simulink model "Timers_Basic"  (R2024a)
settings: Solver=VariableStepAuto  StartTime=0.0  StopTime=10.0  RelTol=1e-3
undefined symbols (not defined in the file or in its folder): DINT, slplc
(part 1 of 2)
settings Model: PacingRate=13  Creator=Jack Vranicar  LastModifiedBy=Jack Vranicar

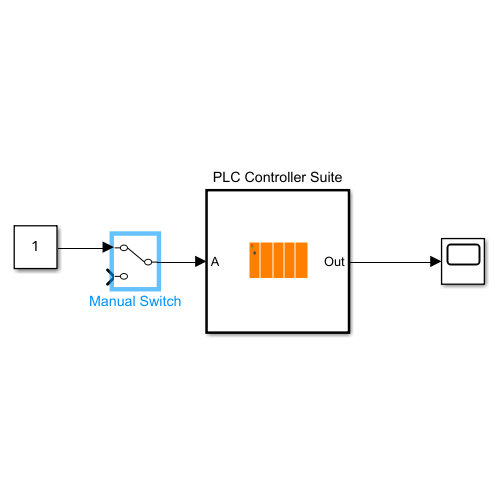
[thumbnail: Simulink's stored preview of the top-level diagram]
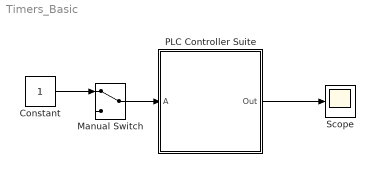
== system Timers_Basic ==
  Constant : Constant  OutDataTypeStr=Inherit: Inherit via back propagation
  Manual Switch : ManualSwitch
  PLC Controller Suite : Subsystem  TreatAsAtomicUnit=on  mask{PLCBlockType=PLCController, PLCPOUType=PLC Controller}
      mask init:
      | slplc.callbacks.initController(gcb);
      settings: OpenFcn=slplc.callbacks.openPOUBlock(gcb);
      mask Help: web([docroot '/plccoder/ref/plccontrollersuite' '.html']);
      mask DialogControl PLCBlockTitle Prompt: PLC Controller Block
  Scope : Scope
  wires:
  Manual Switch/1 -> PLC Controller Suite/1(A)
  Constant/1 -> Manual Switch/1
  PLC Controller Suite/1(Out) -> Scope/1

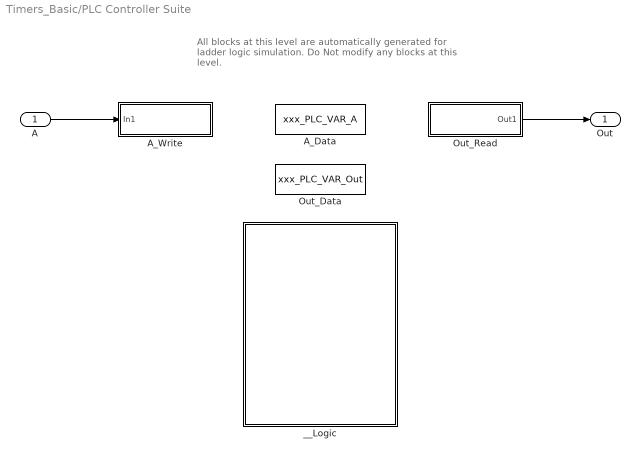
== system Timers_Basic/PLC Controller Suite ==
  note: All blocks at this level are automatically generated for ladder logic simulation.
      | Do Not modify any blocks at this level.
  A : Inport  OutDataTypeStr=boolean
  A_Data : DataStoreMemory  Tag=POUVariable  Priority=10  DataStoreName=xxx_PLC_VAR_A  ShowAdditionalParam=off  OutDataTypeStr=boolean  Dimensions=1
  A_Write : Subsystem  Priority=11  DisableCoverage=on  TreatAsAtomicUnit=on  mask{PLCOperandTag=A, PLCOperandExpression=xxx_PLC_VAR_A, PLCBlockType=VarWrite, PLCPOUType=VarWrite}
      mask prompts: PLCOperandTag "Operand Tag:"
      mask init:
      | slplc.callbacks.initInstruction(gcb);
      mask Help: web([docroot '/plccoder/ref/varwrite' '.html']);
      mask DialogControl PLCBlockTitle Prompt: Variable Write
      mask Display: disp(get_param(gcb, 'PLCOperandTag'));
  Out_Data : DataStoreMemory  Tag=POUVariable  Priority=10  DataStoreName=xxx_PLC_VAR_Out  ShowAdditionalParam=off  OutDataTypeStr=boolean  Dimensions=1
  Out_Read : Subsystem  Priority=13  DisableCoverage=on  TreatAsAtomicUnit=on  mask{PLCOperandTag=Out, PLCOperandExpression=xxx_PLC_VAR_Out, PLCBlockType=VarRead, PLCPOUType=VarRead}
      mask prompts: PLCOperandTag "Operand Tag"
      mask init:
      | block = gcb;
      | maskObj = Simulink.Mask.get(block);
      | maskObj.Display = sprintf('disp(''%s'');', PLCOperandTag);
      | slplc.callbacks.initInstruction(gcb);
      mask Help: web([docroot '/plccoder/ref/varread' '.html']);
      mask DialogControl PLCBlockTitle Prompt: Variable Read
      mask Display: disp('Out');
  __Logic : Subsystem  Priority=12  TreatAsAtomicUnit=on
  Out : Outport
  wires:
  A/1 -> A_Write/1(In1)
  Out_Read/1(Out1) -> Out/1

== system Timers_Basic/PLC Controller Suite/A_Write ==
  In1 : Inport
  __CoreVarWrite : Subsystem  Tag=CoreVarWriteBlock  DisableCoverage=on  TreatAsAtomicUnit=on  mask{PLCBlockType=CoreVarWrite}
      mask init:
      | slplc.callbacks.initCoreVariable(gcb, 'write');
      mask DialogControl PLCBlockTitle Prompt: Core Variable Write
  wires:
  In1/1 -> __CoreVarWrite/1(u)

== system Timers_Basic/PLC Controller Suite/Out_Read ==
  __CoreVarRead : Subsystem  Tag=CoreVarReadBlock  DisableCoverage=on  TreatAsAtomicUnit=on  mask{PLCBlockType=CoreVarRead}
      mask init:
      | slplc.callbacks.initCoreVariable(gcb, 'read');
      mask DialogControl PLCBlockTitle Prompt: Core Variable Read
  Out1 : Outport  VectorParamsAs1DForOutWhenUnconnected=off
  wires:
  __CoreVarRead/1(y) -> Out1/1

== system Timers_Basic/PLC Controller Suite/__Logic ==
  Controller Tags : Subsystem  Tag=ControllerVariableSS  DisableCoverage=on  TreatAsAtomicUnit=on  mask{PLCVarAName=A, PLCVarAAddress=<empty>, PLCVarAMapping=Input Symbol, PLCVarAPortIndex=1, PLCVarADataType=boolean, PLCVarASize=1, PLCVarAInitialValue=0, PLCVarAToDelete=off, PLCVarOutName=Out, PLCVarOutAddress=<empty>, PLCVarOutMapping=Output Symbol, PLCVarOutPortIndex=1, PLCVarOutDataType=boolean, PLCVarOutSize=1, PLCVarOutInitialValue=0, PLCVarOutToDelete=off}
      mask init:
      | slplc.callbacks.initControllerVarSS(gcb);
      settings: OpenFcn=slplc.callbacks.openControllerVariableSS(gcb);
      mask Help: web([docroot '/plccoder/ref/controllertags' '.html']);
      mask TypeOptions PLCVarAMapping: Global Variable | Input Symbol | Output Symbol
      mask Callback PLCVarAMapping: slplc.callbacks.updateControllerVarSS(gcb);
      mask TypeOptions PLCVarAPortIndex: 1 | 2
      mask TypeOptions PLCVarOutMapping: Global Variable | Input Symbol | Output Symbol
      mask Callback PLCVarOutMapping: slplc.callbacks.updateControllerVarSS(gcb);
      mask TypeOptions PLCVarOutPortIndex: 1 | 2
      mask DialogControl PLCBlockTitle Prompt: Global Variable and Symbol Spreadsheet
      mask DialogControl PLCVarListHeaderName Prompt: Name
      mask DialogControl PLCVarListHeaderAddress Prompt: Address (At)
      mask DialogControl PLCVarListHeaderMapping Prompt: Mapping Type
      mask DialogControl PLCVarListHeaderPortIndex Prompt: Port
      mask DialogControl PLCVarListHeaderDataType Prompt: Data Type
      mask DialogControl PLCVarListHeaderSize Prompt: Size
      mask DialogControl PLCVarListHeaderInitialValue Prompt: Initial Value
      mask DialogControl PLCVarListHeaderToDelete Prompt: Delete
  Task : Subsystem  TreatAsAtomicUnit=on  mask{PLCBlockType=Task, PLCPOUType=Task, PLCTaskWatchDog=0}
      settings: OpenFcn=slplc.callbacks.openTaskBlock(gcb);
      mask Help: web([docroot '/plccoder/ref/task' '.html']);
      mask DialogControl PLCBlockTitle Prompt: Task
  Up to Parent POU : Subsystem  DisableCoverage=on  TreatAsAtomicUnit=on  mask{PLCBlockType=OpenParentPOU}
      settings: OpenFcn=slplc.callbacks.openParentPOUBlock(gcb);
      mask Help: web([docroot '/plccoder/ref/uptoparentpou' '.html']);
      mask DialogControl PLCBlockTitle Prompt: Add Single Rung

== system Timers_Basic/PLC Controller Suite/A_Write/__CoreVarWrite ==
  u : Inport
  DataWrite : DataStoreWrite  DataStoreName=xxx_PLC_VAR_A  IndexOptions=Index vector (dialog)  Indices=1  OutputSizes=1
  wires:
  u/1 -> DataWrite/1

== system Timers_Basic/PLC Controller Suite/Out_Read/__CoreVarRead ==
  DataRead : DataStoreRead  DataStoreName=xxx_PLC_VAR_Out  IndexOptions=Index vector (dialog)  Indices=1  OutputSizes=1
  y : Outport  VectorParamsAs1DForOutWhenUnconnected=off
  wires:
  DataRead/1 -> y/1

== system Timers_Basic/PLC Controller Suite/__Logic/Controller Tags ==

== system Timers_Basic/PLC Controller Suite/__Logic/Task ==
  Program : Subsystem  TreatAsAtomicUnit=on  mask{PLCPOUType=Program, PLCPOULanguage=LD, PLCBlockType=LDProgram}
      mask prompts: PLCPOUType "POU Type:"
      mask init:
      | slplc.callbacks.initProgram(gcb);
      settings: OpenFcn=slplc.callbacks.openPOUBlock(gcb);
      mask Help: web([docroot '/plccoder/ref/ldprogram' '.html']);
      mask DialogControl PLCBlockTitle Prompt: Program
      mask DialogControl PLCEditPOU Prompt: Edit POU
      mask DialogControl PLCEditInterface Prompt: Edit Variables
  Up to Parent POU : Subsystem  DisableCoverage=on  TreatAsAtomicUnit=on  mask{PLCBlockType=OpenParentPOU}
      settings: OpenFcn=slplc.callbacks.openParentPOUBlock(gcb);
      mask Help: web([docroot '/plccoder/ref/uptoparentpou' '.html']);
      mask DialogControl PLCBlockTitle Prompt: Add Single Rung

== system Timers_Basic/PLC Controller Suite/__Logic/Up to Parent POU ==

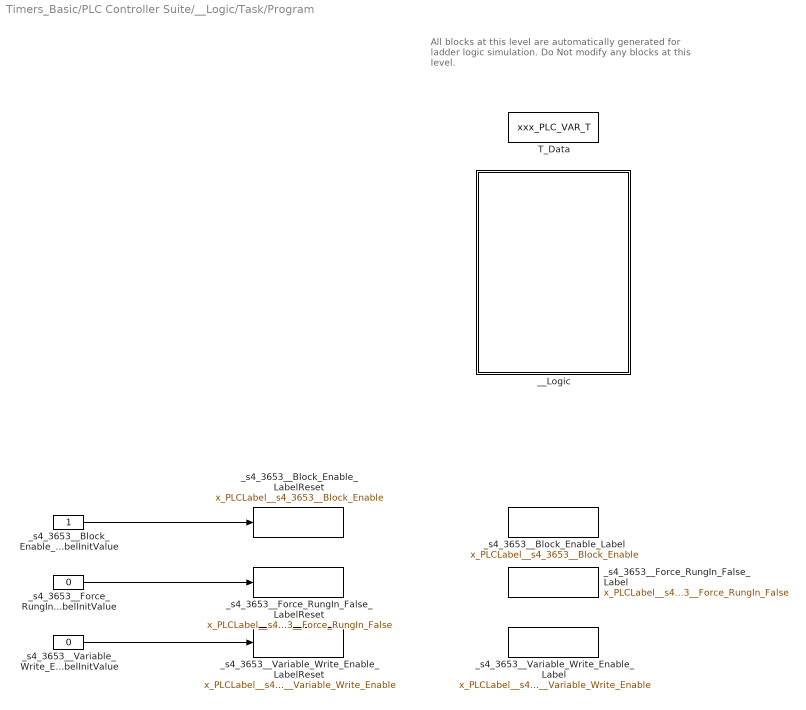
== system Timers_Basic/PLC Controller Suite/__Logic/Task/Program ==
  note: All blocks at this level are automatically generated for ladder logic simulation.
      | Do Not modify any blocks at this level.
  T_Data : DataStoreMemory  Tag=POUVariable  Priority=10  DataStoreName=xxx_PLC_VAR_T  InitialValue=TON_InitialValue  ShowAdditionalParam=off  OutDataTypeStr=Bus: TIMER  Dimensions=1
  __Logic : Subsystem  Priority=12  TreatAsAtomicUnit=on
  _s4_3653__Block_Enable_Label : DataStoreMemory  Priority=10  DataStoreName=x_PLCLabel__s4_3653__Block_Enable  InitialValue=1  ShowAdditionalParam=off  OutDataTypeStr=BOOL  Dimensions=1
  _s4_3653__Block_Enable_LabelInitValue : Constant  OutDataTypeStr=BOOL
  _s4_3653__Block_Enable_LabelReset : DataStoreWrite  Priority=11  DataStoreName=x_PLCLabel__s4_3653__Block_Enable  IndexOptions=Index vector (dialog)  Indices=1  OutputSizes=1
  _s4_3653__Force_RungIn_False_Label : DataStoreMemory  Priority=10  DataStoreName=x_PLCLabel__s4_3653__Force_RungIn_False  ShowAdditionalParam=off  OutDataTypeStr=BOOL  Dimensions=1
  _s4_3653__Force_RungIn_False_LabelInitValue : Constant  Value=0  OutDataTypeStr=BOOL
  _s4_3653__Force_RungIn_False_LabelReset : DataStoreWrite  Priority=11  DataStoreName=x_PLCLabel__s4_3653__Force_RungIn_False  IndexOptions=Index vector (dialog)  Indices=1  OutputSizes=1
  _s4_3653__Variable_Write_Enable_Label : DataStoreMemory  Priority=10  DataStoreName=x_PLCLabel__s4_3653__Variable_Write_Enable  ShowAdditionalParam=off  OutDataTypeStr=BOOL  Dimensions=1
  _s4_3653__Variable_Write_Enable_LabelInitValue : Constant  Value=0  OutDataTypeStr=BOOL
  _s4_3653__Variable_Write_Enable_LabelReset : DataStoreWrite  Priority=11  DataStoreName=x_PLCLabel__s4_3653__Variable_Write_Enable  IndexOptions=Index vector (dialog)  Indices=1  OutputSizes=1
  wires:
  _s4_3653__Block_Enable_LabelInitValue/1 -> _s4_3653__Block_Enable_LabelReset/1
  _s4_3653__Variable_Write_Enable_LabelInitValue/1 -> _s4_3653__Variable_Write_Enable_LabelReset/1
  _s4_3653__Force_RungIn_False_LabelInitValue/1 -> _s4_3653__Force_RungIn_False_LabelReset/1

== system Timers_Basic/PLC Controller Suite/__Logic/Task/Up to Parent POU ==

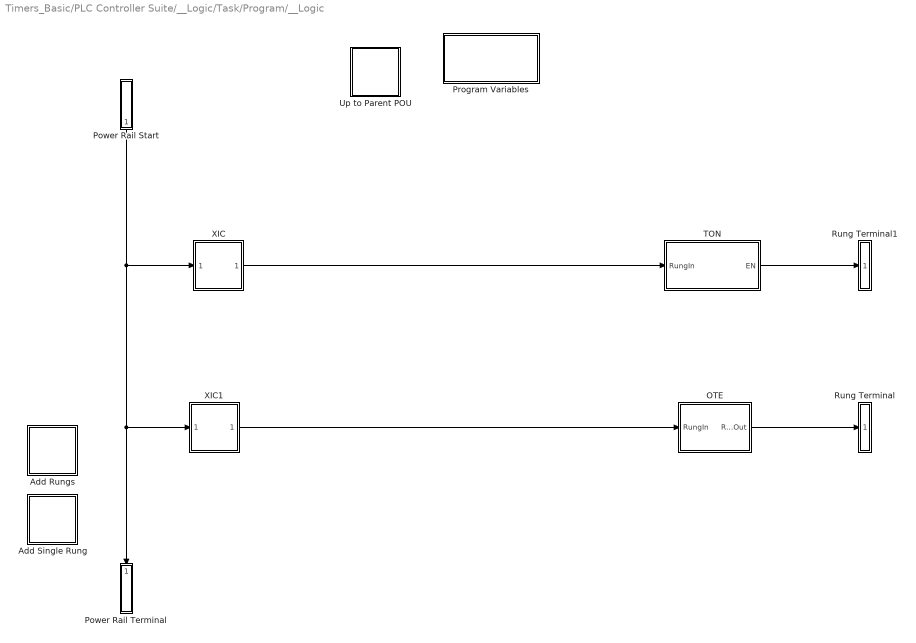
== system Timers_Basic/PLC Controller Suite/__Logic/Task/Program/__Logic ==
  Add Rungs : Subsystem  DisableCoverage=on  TreatAsAtomicUnit=on  mask{PLCRungNumberToAdd=2, PLCBlockType=AddRungs}
      mask prompts: PLCRungNumberToAdd "Rung Number:"
      mask Help: web([docroot '/plccoder/ref/addrungs' '.html']);
      mask DialogControl PLCAddRungs Prompt: Add Rungs
      mask DialogControl PLCRungAddButton Prompt: Add
      mask DialogControl PLCRungAddButton Callback: slplc.callbacks.addLadderRungs(gcb);
      mask Display: disp(sprintf(['Add' newline 'Rungs']));
  Add Single Rung : Subsystem  DisableCoverage=on  TreatAsAtomicUnit=on  mask{PLCRungNumberToAdd=1, PLCBlockType=AddSingleRung}
      settings: OpenFcn=slplc.callbacks.addLadderRungs(gcb);
      mask Help: web([docroot '/plccoder/ref/addsinglerung' '.html']);
      mask DialogControl PLCAddRung Prompt: Add Single Rung
      mask Display: disp(sprintf(['Add' newline '1 Rung']));
  OTE : Subsystem  Priority=6  TreatAsAtomicUnit=on  mask{PLCOperandTag=Out, PLCBlockType=OTE, PLCPOUType=Coil, PLCOperandExpression=xxx_PLC_VAR_Out}
      mask prompts: PLCOperandTag "Operand Tag:"
      mask init:
      | slplc.callbacks.initInstruction(gcb);
      settings: AttributesFormatString=%<PLCOperandTag>
      mask Help: web([docroot '/plccoder/ref/ote' '.html']);
      mask DialogControl PLCBlockTitle Prompt: Output Energize (OTE)
  Power Rail Start : Subsystem  Priority=1  DisableCoverage=on  TreatAsAtomicUnit=on  mask{PLCBlockType=PowerRailStart}
      mask Help: web([docroot '/plccoder/ref/powerrailstart' '.html']);
      mask DialogControl PLCBlockTitle Prompt: Power Rail Start
      mask DialogControl PLCBlockDesc Prompt: This is the ladder diagram left power rail start block.
  Power Rail Terminal : Subsystem  DisableCoverage=on  TreatAsAtomicUnit=on  mask{PLCBlockType=PowerRailTerminal}
      mask Help: web([docroot '/plccoder/ref/powerrailterminal' '.html']);
      mask DialogControl PLCBlockTitle Prompt: Power Rail Terminal
      mask DialogControl PLCBlockDesc Prompt: This is the ladder diagram left power rail terminal block.
  Program Variables : Subsystem  Tag=ProgramVariableSS  DisableCoverage=on  TreatAsAtomicUnit=on  mask{PLCVarTName=T, PLCVarTScope=Local, PLCVarTPortType=Hidden, PLCVarTPortIndex=3, PLCVarTDataType=Bus: TIMER, PLCVarTSize=1, PLCVarTInitialValue=TON_InitialValue, PLCVarTToDelete=off, PLCVarAName=A, PLCVarAScope=External, PLCVarAPortType=Hidden, PLCVarAPortIndex=3, PLCVarADataType=DINT, PLCVarASize=-1, PLCVarAInitialValue=0, PLCVarAToDelete=off, PLCVarOutName=Out, PLCVarOutScope=External, PLCVarOutPortType=Hidden, PLCVarOutPortIndex=3, PLCVarOutDataType=DINT, PLCVarOutSize=-1, PLCVarOutInitialValue=0, PLCVarOutToDelete=off}
      mask init:
      | slplc.callbacks.initPOUVarSS(gcb);
      settings: OpenFcn=slplc.callbacks.openProgramVariableSS(gcb);
      mask Help: web([docroot '/plccoder/ref/programvariables' '.html']);
      mask TypeOptions PLCVarTScope: Local | External
      mask Callback PLCVarTScope: slplc.callbacks.updatePOUVarSS(gcb);
      mask TypeOptions PLCVarTPortType: Hidden | Inport | Outport
      mask Callback PLCVarTPortType: slplc.callbacks.updatePOUVarSS(gcb);
      mask TypeOptions PLCVarTPortIndex: 1 | 2 | 3
      mask TypeOptions PLCVarAScope: Local | External
      mask Callback PLCVarAScope: slplc.callbacks.updatePOUVarSS(gcb);
      mask TypeOptions PLCVarAPortType: Hidden | Inport | Outport
      mask Callback PLCVarAPortType: slplc.callbacks.updatePOUVarSS(gcb);
      mask TypeOptions PLCVarAPortIndex: 1 | 2 | 3
      mask TypeOptions PLCVarOutScope: Local | External
      mask Callback PLCVarOutScope: slplc.callbacks.updatePOUVarSS(gcb);
      mask TypeOptions PLCVarOutPortType: Hidden | Inport | Outport
      mask Callback PLCVarOutPortType: slplc.callbacks.updatePOUVarSS(gcb);
      mask TypeOptions PLCVarOutPortIndex: 1 | 2 | 3
      mask DialogControl PLCBlockTitle Prompt: Program Variable Spreadsheet
      mask DialogControl PLCVarListHeaderName Prompt: Name
      mask DialogControl PLCVarListHeaderScope Prompt: Scope
      mask DialogControl PLCVarListHeaderDataType Prompt: Data Type
      mask DialogControl PLCVarListHeaderSize Prompt: Size
      mask DialogControl PLCVarListHeaderInitialValue Prompt: Initial Value
      mask DialogControl PLCVarListHeaderToDelete Prompt: Delete
  Rung Terminal : Subsystem  Priority=7  DisableCoverage=on  TreatAsAtomicUnit=on  mask{PLCRungTerminalIndex=2, PLCBlockType=RungTerminal}
      settings: AttributesFormatString=Rung %<PLCRungTerminalIndex>
      mask Help: web([docroot '/plccoder/ref/rungterminal' '.html']);
      mask DialogControl PLCBlockTitle Prompt: Rung Terminal
      mask DialogControl PLCBlockDescText Prompt: This is the ladder diagram rung terminal.
  Rung Terminal1 : Subsystem  Priority=4  DisableCoverage=on  TreatAsAtomicUnit=on  mask{PLCRungTerminalIndex=1, PLCBlockType=RungTerminal}
      settings: AttributesFormatString=Rung %<PLCRungTerminalIndex>
      mask Help: web([docroot '/plccoder/ref/rungterminal' '.html']);
      mask DialogControl PLCBlockTitle Prompt: Rung Terminal
      mask DialogControl PLCBlockDescText Prompt: This is the ladder diagram rung terminal.
  TON : Subsystem  Priority=3  TreatAsAtomicUnit=on  mask{PLCOperandTag=T, PLCTimerSampleTime=0.001, PLCBlockType=TON, PLCPOUType=stdFB, PLCOperandAccess=ReadWrite, PLCOperandExpression=xxx_PLC_VAR_T}
      mask prompts: PLCOperandTag "Timer Tag:"; PLCTimerSampleTime "Timer Sample Time:"
      mask init:
      | block = gcb;
      | maskObj = Simulink.Mask.get(block);
      | maskObj.Display = sprintf('disp([''%s'' newline newline ''%s'']);', PLCBlockType, PLCOperandTag);
      | slplc.callbacks.initInstruction(block);
      settings: AttributesFormatString=%<PLCBlockType>: %<PLCOperandTag>
      mask Help: web([docroot '/plccoder/ref/ton' '.html']);
      mask DialogControl PLCBlockTitle Prompt: Timer On Delay (TON)
      mask Display: disp(['TON' newline newline 'T']);
  Up to Parent POU : Subsystem  DisableCoverage=on  TreatAsAtomicUnit=on  mask{PLCBlockType=OpenParentPOU}
      settings: OpenFcn=slplc.callbacks.openParentPOUBlock(gcb);
      mask Help: web([docroot '/plccoder/ref/uptoparentpou' '.html']);
      mask DialogControl PLCBlockTitle Prompt: Add Single Rung
  XIC : Subsystem  Priority=2  TreatAsAtomicUnit=on  mask{PLCOperandTag=A, PLCBlockType=XIC, PLCPOUType=Contact, PLCOperandExpression=xxx_PLC_VAR_A}
      mask prompts: PLCOperandTag "Operand Tag:"
      mask init:
      | slplc.callbacks.initInstruction(gcb);
      settings: AttributesFormatString=%<PLCOperandTag>
      mask Help: web([docroot '/plccoder/ref/xic' '.html']);
      mask DialogControl PLCBlockTitle Prompt: Examine If Closed (XIC)
  XIC1 : Subsystem  Priority=5  TreatAsAtomicUnit=on  mask{PLCOperandTag=T.DN, PLCBlockType=XIC, PLCPOUType=Contact, PLCOperandExpression=xxx_PLC_VAR_T.DN}
      mask prompts: PLCOperandTag "Operand Tag:"
      mask init:
      | slplc.callbacks.initInstruction(gcb);
      settings: AttributesFormatString=%<PLCOperandTag>
      mask Help: web([docroot '/plccoder/ref/xic' '.html']);
      mask DialogControl PLCBlockTitle Prompt: Examine If Closed (XIC)
  wires:
  Power Rail Start/1(PowerOut) -> XIC1/1(RungIn), Power Rail Terminal/1(PowerIn), XIC/1(RungIn)
  XIC/1(RungOut) -> TON/1(RungIn)
  TON/1(EN) -> Rung Terminal1/1(RungIn)
  XIC1/1(RungOut) -> OTE/1(RungIn)
  OTE/1(RungOut) -> Rung Terminal/1(RungIn)

== system Timers_Basic/PLC Controller Suite/__Logic/Task/Program/__Logic/Add Rungs ==

== system Timers_Basic/PLC Controller Suite/__Logic/Task/Program/__Logic/Add Single Rung ==

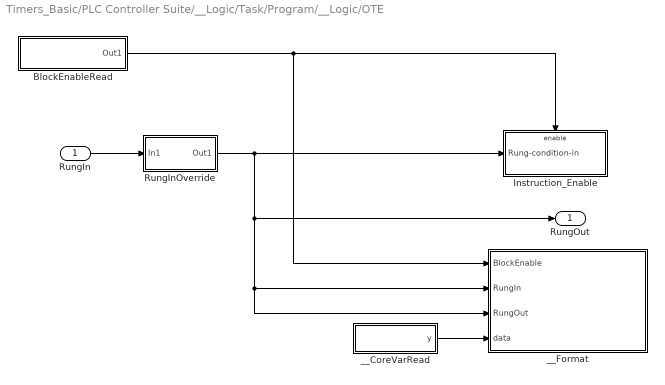
== system Timers_Basic/PLC Controller Suite/__Logic/Task/Program/__Logic/OTE ==
  RungIn : Inport  PortDimensions=1
  BlockEnableRead : Subsystem  DisableCoverage=on  TreatAsAtomicUnit=on  mask{PLCLabelTag=_Block_Enable, PLCBlockType=BlockEnableRead}
      mask prompts: PLCLabelTag "Label Tag:"
      mask init:
      | block = gcb;
      | maskObj = Simulink.Mask.get(block);
      | maskObj.Display = sprintf('disp(''%s'');', PLCLabelTag);
      mask Help: web([docroot '/plccoder/ref/blockenableread' '.html']);
      mask DialogControl PLCBlockTitle Prompt: Block Enable Read
      mask Display: disp('_Block_Enable');
  Instruction_Enable : Subsystem  Priority=12  TreatAsAtomicUnit=on
  RungInOverride : Subsystem  DisableCoverage=on  TreatAsAtomicUnit=on
  __CoreVarRead : Subsystem  Tag=CoreVarReadBlock  DisableCoverage=on  TreatAsAtomicUnit=on  mask{PLCBlockType=CoreVarRead}
      mask init:
      | slplc.callbacks.initCoreVariable(gcb, 'read');
      mask Help: web([docroot '/plccoder/ref/__corevarread' '.html']);
      mask DialogControl PLCBlockTitle Prompt: Core Variable Read
  __Format : MATLAB Function  Tag=PLC_Format_Boolean  Priority=20  DisableCoverage=on  InitFcn=slplc.utils.setBlockAppearance('reset', '%<PLCOperandTag>');  StopFcn=slplc.utils.setBlockAppearance('reset', '%<PLCOperandTag>');  TreatAsAtomicUnit=on
  RungOut : Outport  OutDataTypeStr=BOOL  PortDimensions=1  InitialOutput=false  VectorParamsAs1DForOutWhenUnconnected=off
  wires:
  RungIn/1 -> RungInOverride/1(In1)
  BlockEnableRead/1(Out1) -> __Format/1(BlockEnable), Instruction_Enable/Enable
  RungInOverride/1(Out1) -> __Format/2(RungIn), __Format/3(RungOut), RungOut/1, Instruction_Enable/1(Rung-condition-in)
  __CoreVarRead/1(y) -> __Format/4(data)

== system Timers_Basic/PLC Controller Suite/__Logic/Task/Program/__Logic/Power Rail Start ==
  PLCPowerOn : Constant  Value=true  OutDataTypeStr=BOOL
  __Format : MATLAB Function  Tag=PLC_Format_ENO  Priority=20  DisableCoverage=on  InitFcn=slplc.utils.setBlockAppearance('reset', '', {'black', 'black'});  StopFcn=slplc.utils.setBlockAppearance('reset', '', {'black', 'black'});  TreatAsAtomicUnit=on
  PowerOut : Outport  VectorParamsAs1DForOutWhenUnconnected=off
  wires:
  PLCPowerOn/1 -> __Format/1(RungOut), PowerOut/1

== system Timers_Basic/PLC Controller Suite/__Logic/Task/Program/__Logic/Power Rail Terminal ==
  PowerIn : Inport
  Terminator3 : Terminator
  wires:
  PowerIn/1 -> Terminator3/1

== system Timers_Basic/PLC Controller Suite/__Logic/Task/Program/__Logic/Program Variables ==

== system Timers_Basic/PLC Controller Suite/__Logic/Task/Program/__Logic/Rung Terminal ==
  RungIn : Inport
  Terminator : Terminator
  wires:
  RungIn/1 -> Terminator/1

== system Timers_Basic/PLC Controller Suite/__Logic/Task/Program/__Logic/Rung Terminal1 ==
  RungIn : Inport
  Terminator : Terminator
  wires:
  RungIn/1 -> Terminator/1

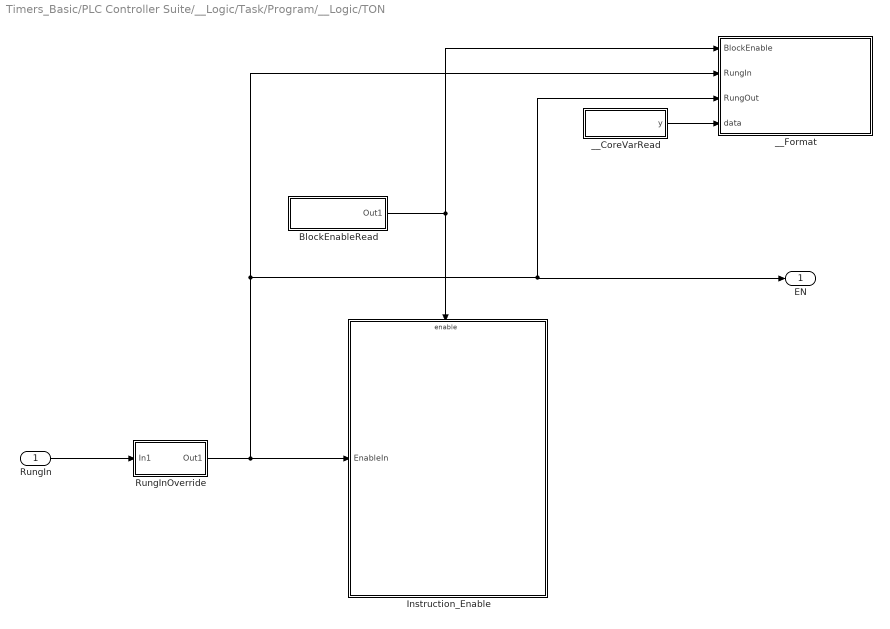
== system Timers_Basic/PLC Controller Suite/__Logic/Task/Program/__Logic/TON ==
  RungIn : Inport
  BlockEnableRead : Subsystem  DisableCoverage=on  TreatAsAtomicUnit=on  mask{PLCLabelTag=_Block_Enable, PLCBlockType=BlockEnableRead}
      mask prompts: PLCLabelTag "Label Tag:"
      mask init:
      | block = gcb;
      | maskObj = Simulink.Mask.get(block);
      | maskObj.Display = sprintf('disp(''%s'');', PLCLabelTag);
      mask Help: web([docroot '/plccoder/ref/blockenableread' '.html']);
      mask DialogControl PLCBlockTitle Prompt: Block Enable Read
      mask Display: disp('_Block_Enable');
  Instruction_Enable : Subsystem  Priority=12
  RungInOverride : Subsystem  DisableCoverage=on  TreatAsAtomicUnit=on
  __CoreVarRead : Subsystem  Tag=CoreVarReadBlock  DisableCoverage=on  TreatAsAtomicUnit=on  mask{PLCBlockType=CoreVarRead}
      mask init:
      | slplc.callbacks.initCoreVariable(gcb, 'read');
      mask Help: web([docroot '/plccoder/ref/__corevarread' '.html']);
      mask DialogControl PLCBlockTitle Prompt: Core Variable Read
  __Format : MATLAB Function  Tag=PLC_Format_FB  Priority=20  DisableCoverage=on  InitFcn=slplc.utils.setBlockAppearance('reset', '%<PLCBlockType>: %<PLCOperandTag>');  StopFcn=slplc.utils.setBlockAppearance('reset', '%<PLCBlockType>: %<PLCOperandTag>');  TreatAsAtomicUnit=on
  EN : Outport  VectorParamsAs1DForOutWhenUnconnected=off
  wires:
  __CoreVarRead/1(y) -> __Format/4(data)
  BlockEnableRead/1(Out1) -> __Format/1(BlockEnable), Instruction_Enable/Enable
  RungIn/1 -> RungInOverride/1(In1)
  RungInOverride/1(Out1) -> __Format/2(RungIn), EN/1, __Format/3(RungOut), Instruction_Enable/1(EnableIn)

== system Timers_Basic/PLC Controller Suite/__Logic/Task/Program/__Logic/Up to Parent POU ==

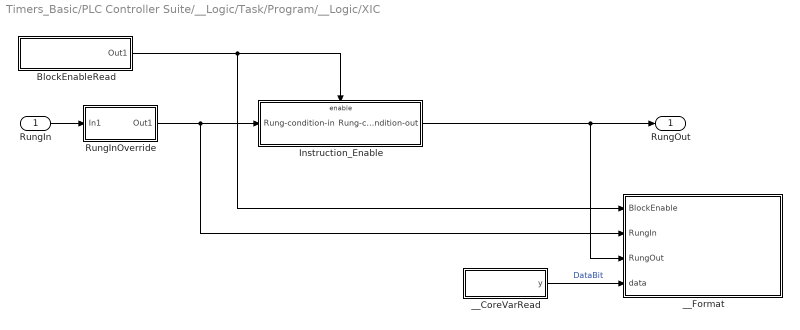
== system Timers_Basic/PLC Controller Suite/__Logic/Task/Program/__Logic/XIC ==
  RungIn : Inport  PortDimensions=1
  BlockEnableRead : Subsystem  DisableCoverage=on  TreatAsAtomicUnit=on  mask{PLCLabelTag=_Block_Enable, PLCBlockType=BlockEnableRead}
      mask prompts: PLCLabelTag "Label Tag:"
      mask init:
      | block = gcb;
      | maskObj = Simulink.Mask.get(block);
      | maskObj.Display = sprintf('disp(''%s'');', PLCLabelTag);
      mask Help: web([docroot '/plccoder/ref/blockenableread' '.html']);
      mask DialogControl PLCBlockTitle Prompt: Block Enable Read
      mask Display: disp('_Block_Enable');
  Instruction_Enable : Subsystem  Priority=12  TreatAsAtomicUnit=on
  RungInOverride : Subsystem  DisableCoverage=on  TreatAsAtomicUnit=on
  __CoreVarRead : Subsystem  Tag=CoreVarReadBlock  DisableCoverage=on  TreatAsAtomicUnit=on  mask{PLCBlockType=CoreVarRead}
      mask init:
      | slplc.callbacks.initCoreVariable(gcb, 'read');
      mask Help: web([docroot '/plccoder/ref/__corevarread' '.html']);
      mask DialogControl PLCBlockTitle Prompt: Core Variable Read
  __Format : MATLAB Function  Tag=PLC_Format_Boolean  Priority=20  DisableCoverage=on  InitFcn=slplc.utils.setBlockAppearance('reset', '%<PLCOperandTag>');  StopFcn=slplc.utils.setBlockAppearance('reset', '%<PLCOperandTag>');  TreatAsAtomicUnit=on
  RungOut : Outport  OutDataTypeStr=BOOL  PortDimensions=1  InitialOutput=false  VectorParamsAs1DForOutWhenUnconnected=off
  wires:
  __CoreVarRead/1(y) -> __Format/4(data)  "DataBit"
  RungInOverride/1(Out1) -> Instruction_Enable/1(Rung-condition-in), __Format/2(RungIn)
  BlockEnableRead/1(Out1) -> Instruction_Enable/Enable, __Format/1(BlockEnable)
  Instruction_Enable/1(Rung-condition-out) -> RungOut/1, __Format/3(RungOut)
  RungIn/1 -> RungInOverride/1(In1)

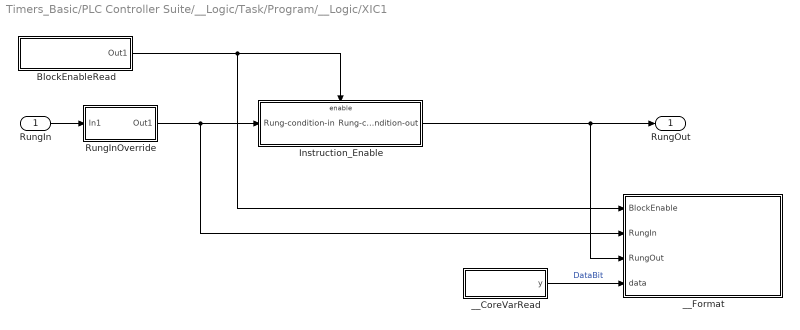
== system Timers_Basic/PLC Controller Suite/__Logic/Task/Program/__Logic/XIC1 ==
  RungIn : Inport  PortDimensions=1
  BlockEnableRead : Subsystem  DisableCoverage=on  TreatAsAtomicUnit=on  mask{PLCLabelTag=_Block_Enable, PLCBlockType=BlockEnableRead}
      mask prompts: PLCLabelTag "Label Tag:"
      mask init:
      | block = gcb;
      | maskObj = Simulink.Mask.get(block);
      | maskObj.Display = sprintf('disp(''%s'');', PLCLabelTag);
      mask Help: web([docroot '/plccoder/ref/blockenableread' '.html']);
      mask DialogControl PLCBlockTitle Prompt: Block Enable Read
      mask Display: disp('_Block_Enable');
  Instruction_Enable : Subsystem  Priority=12  TreatAsAtomicUnit=on
  RungInOverride : Subsystem  DisableCoverage=on  TreatAsAtomicUnit=on
  __CoreVarRead : Subsystem  Tag=CoreVarReadBlock  DisableCoverage=on  TreatAsAtomicUnit=on  mask{PLCBlockType=CoreVarRead}
      mask init:
      | slplc.callbacks.initCoreVariable(gcb, 'read');
      mask Help: web([docroot '/plccoder/ref/__corevarread' '.html']);
      mask DialogControl PLCBlockTitle Prompt: Core Variable Read
  __Format : MATLAB Function  Tag=PLC_Format_Boolean  Priority=20  DisableCoverage=on  InitFcn=slplc.utils.setBlockAppearance('reset', '%<PLCOperandTag>');  StopFcn=slplc.utils.setBlockAppearance('reset', '%<PLCOperandTag>');  TreatAsAtomicUnit=on
  RungOut : Outport  OutDataTypeStr=BOOL  PortDimensions=1  InitialOutput=false  VectorParamsAs1DForOutWhenUnconnected=off
  wires:
  __CoreVarRead/1(y) -> __Format/4(data)  "DataBit"
  RungInOverride/1(Out1) -> Instruction_Enable/1(Rung-condition-in), __Format/2(RungIn)
  BlockEnableRead/1(Out1) -> Instruction_Enable/Enable, __Format/1(BlockEnable)
  Instruction_Enable/1(Rung-condition-out) -> RungOut/1, __Format/3(RungOut)
  RungIn/1 -> RungInOverride/1(In1)

== system Timers_Basic/PLC Controller Suite/__Logic/Task/Program/__Logic/OTE/BlockEnableRead ==
  __CoreLabelRead : Subsystem  Tag=CoreVarReadBlock  DisableCoverage=on  TreatAsAtomicUnit=on  mask{PLCBlockType=CoreLabelRead}
      mask init:
      | slplc.callbacks.initRoutineLabelRead(gcb);
      mask Help: web([docroot '/plccoder/ref/__corelabelread' '.html']);
      mask DialogControl PLCBlockTitle Prompt: Core Label Read
  Out1 : Outport  VectorParamsAs1DForOutWhenUnconnected=off
  wires:
  __CoreLabelRead/1(Out1) -> Out1/1

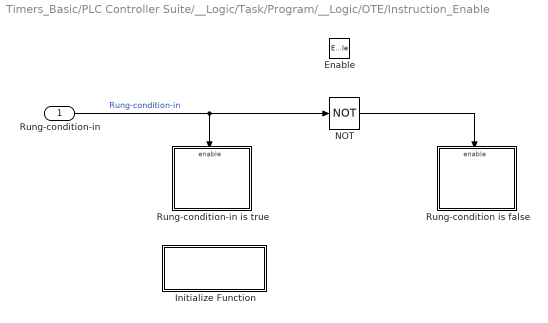
== system Timers_Basic/PLC Controller Suite/__Logic/Task/Program/__Logic/OTE/Instruction_Enable ==
  Rung-condition-in : Inport  OutDataTypeStr=BOOL
  Enable : EnablePort
  Initialize Function : Subsystem  TreatAsAtomicUnit=on
  NOT : Logic  Operator=NOT  IconShape=distinctive  AllPortsSameDT=off  OutDataTypeStr=boolean
  Rung-condition is false : Subsystem  Priority=12  DisableCoverage=on
  Rung-condition-in is true : Subsystem  Priority=12  DisableCoverage=on
  wires:
  NOT/1 -> Rung-condition is false/Enable
  Rung-condition-in/1 -> Rung-condition-in is true/Enable, NOT/1  "Rung-condition-in"

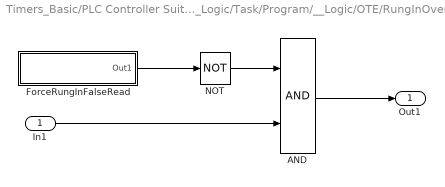
== system Timers_Basic/PLC Controller Suite/__Logic/Task/Program/__Logic/OTE/RungInOverride ==
  In1 : Inport
  AND : Logic  AllPortsSameDT=off  OutDataTypeStr=boolean
  ForceRungInFalseRead : Subsystem  DisableCoverage=on  TreatAsAtomicUnit=on  mask{PLCLabelTag=_Force_RungIn_False, PLCBlockType=ForceRungInFalseRead}
      mask prompts: PLCLabelTag "Label Tag:"
      mask init:
      | block = gcb;
      | maskObj = Simulink.Mask.get(block);
      | maskObj.Display = sprintf('disp(''%s'');', PLCLabelTag);
      mask Help: web([docroot '/plccoder/ref/forcerunginfalseread' '.html']);
      mask DialogControl PLCBlockTitle Prompt: Force Rung-In False Read
      mask Display: disp('_Force_RungIn_False');
  NOT : Logic  Operator=NOT  IconShape=distinctive  AllPortsSameDT=off  OutDataTypeStr=boolean
  Out1 : Outport  VectorParamsAs1DForOutWhenUnconnected=off
  wires:
  AND/1 -> Out1/1
  In1/1 -> AND/2
  ForceRungInFalseRead/1(Out1) -> NOT/1
  NOT/1 -> AND/1

== system Timers_Basic/PLC Controller Suite/__Logic/Task/Program/__Logic/OTE/__CoreVarRead ==
  DataRead : DataStoreRead  DataStoreName=xxx_PLC_VAR_Out  IndexOptions=Index vector (dialog)  Indices=1  OutputSizes=1
  y : Outport  VectorParamsAs1DForOutWhenUnconnected=off
  wires:
  DataRead/1 -> y/1

== system Timers_Basic/PLC Controller Suite/__Logic/Task/Program/__Logic/TON/BlockEnableRead ==
  __CoreLabelRead : Subsystem  Tag=CoreVarReadBlock  DisableCoverage=on  TreatAsAtomicUnit=on  mask{PLCBlockType=CoreLabelRead}
      mask init:
      | slplc.callbacks.initRoutineLabelRead(gcb);
      mask Help: web([docroot '/plccoder/ref/__corelabelread' '.html']);
      mask DialogControl PLCBlockTitle Prompt: Core Label Read
  Out1 : Outport  VectorParamsAs1DForOutWhenUnconnected=off
  wires:
  __CoreLabelRead/1(Out1) -> Out1/1

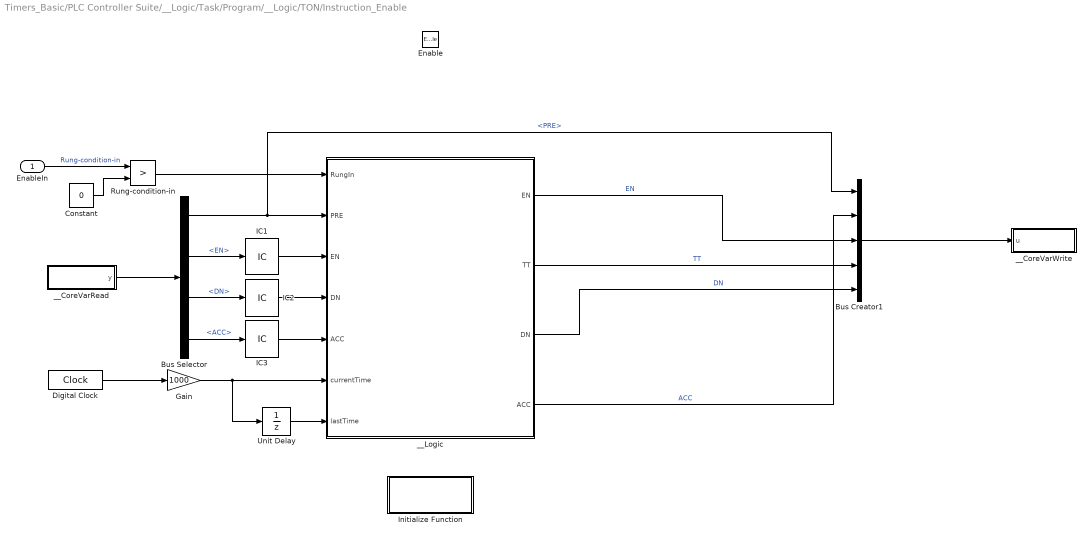
== system Timers_Basic/PLC Controller Suite/__Logic/Task/Program/__Logic/TON/Instruction_Enable ==
  EnableIn : Inport
  Enable : EnablePort
  Bus Creator1 : BusCreator  Inputs=5  OutDataTypeStr=Bus: TIMER  NonVirtualBus=on
  Bus Selector : BusSelector  OutputSignals=PRE,EN,DN,ACC
  Constant : Constant  Value=0
  Digital Clock : DigitalClock  SampleTime=PLCTimerSampleTime
  Gain : Gain  Gain=1000
  IC1 : InitialCondition  Value=false
  IC2 : InitialCondition  Value=false
  IC3 : InitialCondition  Value=0
  Initialize Function : Subsystem  TreatAsAtomicUnit=on
  Rung-condition-in : RelationalOperator  Operator=>  OutDataTypeStr=boolean  RndMeth=Simplest  InputSameDT=off
  Unit Delay : UnitDelay  SampleTime=-1  HasFrameUpgradeWarning=on
  __CoreVarRead : Subsystem  Tag=CoreVarReadBlock  DisableCoverage=on  TreatAsAtomicUnit=on  mask{PLCBlockType=CoreVarRead}
      mask init:
      | slplc.callbacks.initCoreVariable(gcb, 'read');
      mask Help: web([docroot '/plccoder/ref/__corevarread' '.html']);
      mask DialogControl PLCBlockTitle Prompt: Core Variable Read
  __CoreVarWrite : Subsystem  Tag=CoreVarWriteBlock  DisableCoverage=on  TreatAsAtomicUnit=on  mask{PLCBlockType=CoreVarWrite}
      mask init:
      | slplc.callbacks.initCoreVariable(gcb, 'write');
      mask Help: web([docroot '/plccoder/ref/__corevarwrite' '.html']);
      mask DialogControl PLCBlockTitle Prompt: Core Variable Write
  __Logic : MATLAB Function  Priority=12  DisableCoverage=on
  wires:
  IC3/1 -> __Logic/5("ACC ")
  IC2/1 -> __Logic/4("DN ")
  IC1/1 -> __Logic/3("EN ")
  Rung-condition-in/1 -> __Logic/1(RungIn)
  Bus Selector/2 -> IC1/1  "<EN>"
  Gain/1 -> __Logic/6(currentTime), Unit Delay/1
  Bus Selector/3 -> IC2/1  "<DN>"
  __CoreVarRead/1(y) -> Bus Selector/1
  Unit Delay/1 -> __Logic/7(lastTime)
  Bus Creator1/1 -> __CoreVarWrite/1(u)
  __Logic/4(ACC) -> Bus Creator1/2  "ACC"
  __Logic/3(DN) -> Bus Creator1/5  "DN"
  Digital Clock/1 -> Gain/1
  EnableIn/1 -> Rung-condition-in/1  "Rung-condition-in"
  Bus Selector/1 -> Bus Creator1/1, __Logic/2(PRE)  "<PRE>"
  __Logic/2(TT) -> Bus Creator1/4  "TT"
  Bus Selector/4 -> IC3/1  "<ACC>"
  __Logic/1(EN) -> Bus Creator1/3  "EN"
  Constant/1 -> Rung-condition-in/2

== system Timers_Basic/PLC Controller Suite/__Logic/Task/Program/__Logic/TON/RungInOverride ==
  In1 : Inport
  AND : Logic  AllPortsSameDT=off  OutDataTypeStr=boolean
  ForceRungInFalseRead : Subsystem  DisableCoverage=on  TreatAsAtomicUnit=on  mask{PLCLabelTag=_Force_RungIn_False, PLCBlockType=ForceRungInFalseRead}
      mask prompts: PLCLabelTag "Label Tag:"
      mask init:
      | block = gcb;
      | maskObj = Simulink.Mask.get(block);
      | maskObj.Display = sprintf('disp(''%s'');', PLCLabelTag);
      mask Help: web([docroot '/plccoder/ref/forcerunginfalseread' '.html']);
      mask DialogControl PLCBlockTitle Prompt: Force Rung-In False Read
      mask Display: disp('_Force_RungIn_False');
  NOT : Logic  Operator=NOT  IconShape=distinctive  AllPortsSameDT=off  OutDataTypeStr=boolean
  Out1 : Outport  VectorParamsAs1DForOutWhenUnconnected=off
  wires:
  AND/1 -> Out1/1
  In1/1 -> AND/2
  ForceRungInFalseRead/1(Out1) -> NOT/1
  NOT/1 -> AND/1

== system Timers_Basic/PLC Controller Suite/__Logic/Task/Program/__Logic/TON/__CoreVarRead ==
  DataRead : DataStoreRead  DataStoreName=xxx_PLC_VAR_T  IndexOptions=Index vector (dialog)  Indices=1  OutputSizes=1
  y : Outport  VectorParamsAs1DForOutWhenUnconnected=off
  wires:
  DataRead/1 -> y/1

== system Timers_Basic/PLC Controller Suite/__Logic/Task/Program/__Logic/XIC/BlockEnableRead ==
  __CoreLabelRead : Subsystem  Tag=CoreVarReadBlock  DisableCoverage=on  TreatAsAtomicUnit=on  mask{PLCBlockType=CoreLabelRead}
      mask init:
      | slplc.callbacks.initRoutineLabelRead(gcb);
      mask Help: web([docroot '/plccoder/ref/__corelabelread' '.html']);
      mask DialogControl PLCBlockTitle Prompt: Core Label Read
  Out1 : Outport  VectorParamsAs1DForOutWhenUnconnected=off
  wires:
  __CoreLabelRead/1(Out1) -> Out1/1

== system Timers_Basic/PLC Controller Suite/__Logic/Task/Program/__Logic/XIC/Instruction_Enable ==
  Rung-condition-in : Inport  OutDataTypeStr=BOOL
  Enable : EnablePort
  Logical Operator : Logic  OutDataTypeStr=BOOL
  __CoreVarRead : Subsystem  Tag=CoreVarReadBlock  DisableCoverage=on  TreatAsAtomicUnit=on  mask{PLCBlockType=CoreVarRead}
      mask init:
      | slplc.callbacks.initCoreVariable(gcb, 'read');
      mask Help: web([docroot '/plccoder/ref/__corevarread' '.html']);
      mask DialogControl PLCBlockTitle Prompt: Core Variable Read
  Rung-condition-out : Outport  VectorParamsAs1DForOutWhenUnconnected=off
  wires:
  Rung-condition-in/1 -> Logical Operator/1  "Rung-condition-in"
  Logical Operator/1 -> Rung-condition-out/1  "Rung-condition-out"
  __CoreVarRead/1(y) -> Logical Operator/2  "DataBit"

== system Timers_Basic/PLC Controller Suite/__Logic/Task/Program/__Logic/XIC/RungInOverride ==
  In1 : Inport
  AND : Logic  AllPortsSameDT=off  OutDataTypeStr=boolean
  ForceRungInFalseRead : Subsystem  DisableCoverage=on  TreatAsAtomicUnit=on  mask{PLCLabelTag=_Force_RungIn_False, PLCBlockType=ForceRungInFalseRead}
      mask prompts: PLCLabelTag "Label Tag:"
      mask init:
      | block = gcb;
      | maskObj = Simulink.Mask.get(block);
      | maskObj.Display = sprintf('disp(''%s'');', PLCLabelTag);
      mask Help: web([docroot '/plccoder/ref/forcerunginfalseread' '.html']);
      mask DialogControl PLCBlockTitle Prompt: Force Rung-In False Read
      mask Display: disp('_Force_RungIn_False');
  NOT : Logic  Operator=NOT  IconShape=distinctive  AllPortsSameDT=off  OutDataTypeStr=boolean
  Out1 : Outport  VectorParamsAs1DForOutWhenUnconnected=off
  wires:
  AND/1 -> Out1/1
  In1/1 -> AND/2
  ForceRungInFalseRead/1(Out1) -> NOT/1
  NOT/1 -> AND/1

== system Timers_Basic/PLC Controller Suite/__Logic/Task/Program/__Logic/XIC/__CoreVarRead ==
  DataRead : DataStoreRead  DataStoreName=xxx_PLC_VAR_A  IndexOptions=Index vector (dialog)  Indices=1  OutputSizes=1
  y : Outport  VectorParamsAs1DForOutWhenUnconnected=off
  wires:
  DataRead/1 -> y/1

== system Timers_Basic/PLC Controller Suite/__Logic/Task/Program/__Logic/XIC1/BlockEnableRead ==
  __CoreLabelRead : Subsystem  Tag=CoreVarReadBlock  DisableCoverage=on  TreatAsAtomicUnit=on  mask{PLCBlockType=CoreLabelRead}
      mask init:
      | slplc.callbacks.initRoutineLabelRead(gcb);
      mask Help: web([docroot '/plccoder/ref/__corelabelread' '.html']);
      mask DialogControl PLCBlockTitle Prompt: Core Label Read
  Out1 : Outport  VectorParamsAs1DForOutWhenUnconnected=off
  wires:
  __CoreLabelRead/1(Out1) -> Out1/1

== system Timers_Basic/PLC Controller Suite/__Logic/Task/Program/__Logic/XIC1/Instruction_Enable ==
  Rung-condition-in : Inport  OutDataTypeStr=BOOL
  Enable : EnablePort
  Logical Operator : Logic  OutDataTypeStr=BOOL
  __CoreVarRead : Subsystem  Tag=CoreVarReadBlock  DisableCoverage=on  TreatAsAtomicUnit=on  mask{PLCBlockType=CoreVarRead}
      mask init:
      | slplc.callbacks.initCoreVariable(gcb, 'read');
      mask Help: web([docroot '/plccoder/ref/__corevarread' '.html']);
      mask DialogControl PLCBlockTitle Prompt: Core Variable Read
  Rung-condition-out : Outport  VectorParamsAs1DForOutWhenUnconnected=off
  wires:
  Rung-condition-in/1 -> Logical Operator/1  "Rung-condition-in"
  Logical Operator/1 -> Rung-condition-out/1  "Rung-condition-out"
  __CoreVarRead/1(y) -> Logical Operator/2  "DataBit"

== system Timers_Basic/PLC Controller Suite/__Logic/Task/Program/__Logic/XIC1/RungInOverride ==
  In1 : Inport
  AND : Logic  AllPortsSameDT=off  OutDataTypeStr=boolean
  ForceRungInFalseRead : Subsystem  DisableCoverage=on  TreatAsAtomicUnit=on  mask{PLCLabelTag=_Force_RungIn_False, PLCBlockType=ForceRungInFalseRead}
      mask prompts: PLCLabelTag "Label Tag:"
      mask init:
      | block = gcb;
      | maskObj = Simulink.Mask.get(block);
      | maskObj.Display = sprintf('disp(''%s'');', PLCLabelTag);
      mask Help: web([docroot '/plccoder/ref/forcerunginfalseread' '.html']);
      mask DialogControl PLCBlockTitle Prompt: Force Rung-In False Read
      mask Display: disp('_Force_RungIn_False');
  NOT : Logic  Operator=NOT  IconShape=distinctive  AllPortsSameDT=off  OutDataTypeStr=boolean
  Out1 : Outport  VectorParamsAs1DForOutWhenUnconnected=off
  wires:
  AND/1 -> Out1/1
  In1/1 -> AND/2
  ForceRungInFalseRead/1(Out1) -> NOT/1
  NOT/1 -> AND/1

== system Timers_Basic/PLC Controller Suite/__Logic/Task/Program/__Logic/XIC1/__CoreVarRead ==
  DataRead : DataStoreRead  DataStoreName=xxx_PLC_VAR_T  DataStoreElements=xxx_PLC_VAR_T.DN  IndexOptions=Index vector (dialog)  Indices=1  OutputSizes=1
  y : Outport  VectorParamsAs1DForOutWhenUnconnected=off
  wires:
  DataRead/1 -> y/1

== system Timers_Basic/PLC Controller Suite/__Logic/Task/Program/__Logic/OTE/BlockEnableRead/__CoreLabelRead ==
  DataRead : DataStoreRead  DataStoreName=x_PLCLabel__s4_3653__Block_Enable  IndexOptions=Index vector (dialog)  Indices=1  OutputSizes=1
  Out1 : Outport  VectorParamsAs1DForOutWhenUnconnected=off
  wires:
  DataRead/1 -> Out1/1

== system Timers_Basic/PLC Controller Suite/__Logic/Task/Program/__Logic/OTE/Instruction_Enable/Initialize Function ==
  Constant : Constant  Value=0  OutDataTypeStr=BOOL
  Event Listener : EventListener  DisableCoverage=on  EventName=reset
  __CoreVarWrite : Subsystem  Tag=CoreVarWriteBlock  DisableCoverage=on  TreatAsAtomicUnit=on  mask{PLCBlockType=CoreVarWrite}
      mask init:
      | slplc.callbacks.initCoreVariable(gcb, 'write');
      mask Help: web([docroot '/plccoder/ref/__corevarwrite' '.html']);
      mask DialogControl PLCBlockTitle Prompt: Core Variable Write
  wires:
  Constant/1 -> __CoreVarWrite/1(u)

== system Timers_Basic/PLC Controller Suite/__Logic/Task/Program/__Logic/OTE/Instruction_Enable/Rung-condition is false ==
  Enable : EnablePort
  Constant : Constant  Value=0  OutDataTypeStr=BOOL
  __CoreVarWrite : Subsystem  Tag=CoreVarWriteBlock  DisableCoverage=on  TreatAsAtomicUnit=on  mask{PLCBlockType=CoreVarWrite}
      mask init:
      | slplc.callbacks.initCoreVariable(gcb, 'write');
      mask Help: web([docroot '/plccoder/ref/__corevarwrite' '.html']);
      mask DialogControl PLCBlockTitle Prompt: Core Variable Write
  wires:
  Constant/1 -> __CoreVarWrite/1(u)

== system Timers_Basic/PLC Controller Suite/__Logic/Task/Program/__Logic/OTE/Instruction_Enable/Rung-condition-in is true ==
  Enable : EnablePort
  Constant : Constant  OutDataTypeStr=BOOL
  __CoreVarWrite : Subsystem  Tag=CoreVarWriteBlock  DisableCoverage=on  TreatAsAtomicUnit=on  mask{PLCBlockType=CoreVarWrite}
      mask init:
      | slplc.callbacks.initCoreVariable(gcb, 'write');
      mask Help: web([docroot '/plccoder/ref/__corevarwrite' '.html']);
      mask DialogControl PLCBlockTitle Prompt: Core Variable Write
  wires:
  Constant/1 -> __CoreVarWrite/1(u)

== system Timers_Basic/PLC Controller Suite/__Logic/Task/Program/__Logic/OTE/RungInOverride/ForceRungInFalseRead ==
  __CoreLabelRead : Subsystem  Tag=CoreVarReadBlock  DisableCoverage=on  TreatAsAtomicUnit=on  mask{PLCBlockType=CoreLabelRead}
      mask init:
      | slplc.callbacks.initRoutineLabelRead(gcb);
      mask Help: web([docroot '/plccoder/ref/__corelabelread' '.html']);
      mask DialogControl PLCBlockTitle Prompt: Core Label Read
  Out1 : Outport  VectorParamsAs1DForOutWhenUnconnected=off
  wires:
  __CoreLabelRead/1(Out1) -> Out1/1

== system Timers_Basic/PLC Controller Suite/__Logic/Task/Program/__Logic/TON/BlockEnableRead/__CoreLabelRead ==
  DataRead : DataStoreRead  DataStoreName=x_PLCLabel__s4_3653__Block_Enable  IndexOptions=Index vector (dialog)  Indices=1  OutputSizes=1
  Out1 : Outport  VectorParamsAs1DForOutWhenUnconnected=off
  wires:
  DataRead/1 -> Out1/1

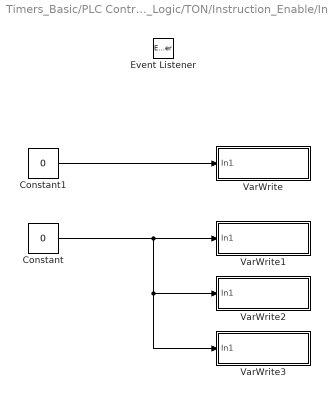
== system Timers_Basic/PLC Controller Suite/__Logic/Task/Program/__Logic/TON/Instruction_Enable/Initialize Function ==
  Constant : Constant  Value=0  OutDataTypeStr=BOOL
  Constant1 : Constant  Value=0  OutDataTypeStr=DINT
  Event Listener : EventListener  DisableCoverage=on  EventName=reset
  VarWrite : Subsystem  DisableCoverage=on  TreatAsAtomicUnit=on  mask{PLCOperandTag=ACC, PLCOperandExpression=xxx_PLC_VAR_T.ACC, PLCBlockType=VarWrite, PLCPOUType=VarWrite}
      mask prompts: PLCOperandTag "Operand Tag:"
      mask init:
      | slplc.callbacks.initInstruction(gcb);
      mask Help: web([docroot '/plccoder/ref/varwrite' '.html']);
      mask DialogControl PLCBlockTitle Prompt: Variable Write
      mask Display: disp(get_param(gcb, 'PLCOperandTag'));
  VarWrite1 : Subsystem  DisableCoverage=on  TreatAsAtomicUnit=on  mask{PLCOperandTag=EN, PLCOperandExpression=xxx_PLC_VAR_T.EN, PLCBlockType=VarWrite, PLCPOUType=VarWrite}
      mask prompts: PLCOperandTag "Operand Tag:"
      mask init:
      | slplc.callbacks.initInstruction(gcb);
      mask Help: web([docroot '/plccoder/ref/varwrite' '.html']);
      mask DialogControl PLCBlockTitle Prompt: Variable Write
      mask Display: disp(get_param(gcb, 'PLCOperandTag'));
  VarWrite2 : Subsystem  DisableCoverage=on  TreatAsAtomicUnit=on  mask{PLCOperandTag=TT, PLCOperandExpression=xxx_PLC_VAR_T.TT, PLCBlockType=VarWrite, PLCPOUType=VarWrite}
      mask prompts: PLCOperandTag "Operand Tag:"
      mask init:
      | slplc.callbacks.initInstruction(gcb);
      mask Help: web([docroot '/plccoder/ref/varwrite' '.html']);
      mask DialogControl PLCBlockTitle Prompt: Variable Write
      mask Display: disp(get_param(gcb, 'PLCOperandTag'));
  VarWrite3 : Subsystem  DisableCoverage=on  TreatAsAtomicUnit=on  mask{PLCOperandTag=DN, PLCOperandExpression=xxx_PLC_VAR_T.DN, PLCBlockType=VarWrite, PLCPOUType=VarWrite}
      mask prompts: PLCOperandTag "Operand Tag:"
      mask init:
      | slplc.callbacks.initInstruction(gcb);
      mask Help: web([docroot '/plccoder/ref/varwrite' '.html']);
      mask DialogControl PLCBlockTitle Prompt: Variable Write
      mask Display: disp(get_param(gcb, 'PLCOperandTag'));
  wires:
  Constant/1 -> VarWrite1/1(In1), VarWrite2/1(In1), VarWrite3/1(In1)
  Constant1/1 -> VarWrite/1(In1)

== system Timers_Basic/PLC Controller Suite/__Logic/Task/Program/__Logic/TON/Instruction_Enable/__CoreVarRead ==
  DataRead : DataStoreRead  DataStoreName=xxx_PLC_VAR_T  IndexOptions=Index vector (dialog)  Indices=1  OutputSizes=1
  y : Outport  VectorParamsAs1DForOutWhenUnconnected=off
  wires:
  DataRead/1 -> y/1

== system Timers_Basic/PLC Controller Suite/__Logic/Task/Program/__Logic/TON/Instruction_Enable/__CoreVarWrite ==
  u : Inport
  DataWrite : DataStoreWrite  DataStoreName=xxx_PLC_VAR_T  IndexOptions=Index vector (dialog)  Indices=1  OutputSizes=1
  wires:
  u/1 -> DataWrite/1

== system Timers_Basic/PLC Controller Suite/__Logic/Task/Program/__Logic/TON/RungInOverride/ForceRungInFalseRead ==
  __CoreLabelRead : Subsystem  Tag=CoreVarReadBlock  DisableCoverage=on  TreatAsAtomicUnit=on  mask{PLCBlockType=CoreLabelRead}
      mask init:
      | slplc.callbacks.initRoutineLabelRead(gcb);
      mask Help: web([docroot '/plccoder/ref/__corelabelread' '.html']);
      mask DialogControl PLCBlockTitle Prompt: Core Label Read
  Out1 : Outport  VectorParamsAs1DForOutWhenUnconnected=off
  wires:
  __CoreLabelRead/1(Out1) -> Out1/1

== system Timers_Basic/PLC Controller Suite/__Logic/Task/Program/__Logic/XIC/BlockEnableRead/__CoreLabelRead ==
  DataRead : DataStoreRead  DataStoreName=x_PLCLabel__s4_3653__Block_Enable  IndexOptions=Index vector (dialog)  Indices=1  OutputSizes=1
  Out1 : Outport  VectorParamsAs1DForOutWhenUnconnected=off
  wires:
  DataRead/1 -> Out1/1

== system Timers_Basic/PLC Controller Suite/__Logic/Task/Program/__Logic/XIC/Instruction_Enable/__CoreVarRead ==
  DataRead : DataStoreRead  DataStoreName=xxx_PLC_VAR_A  IndexOptions=Index vector (dialog)  Indices=1  OutputSizes=1
  y : Outport  VectorParamsAs1DForOutWhenUnconnected=off
  wires:
  DataRead/1 -> y/1

== system Timers_Basic/PLC Controller Suite/__Logic/Task/Program/__Logic/XIC/RungInOverride/ForceRungInFalseRead ==
  __CoreLabelRead : Subsystem  Tag=CoreVarReadBlock  DisableCoverage=on  TreatAsAtomicUnit=on  mask{PLCBlockType=CoreLabelRead}
      mask init:
      | slplc.callbacks.initRoutineLabelRead(gcb);
      mask Help: web([docroot '/plccoder/ref/__corelabelread' '.html']);
      mask DialogControl PLCBlockTitle Prompt: Core Label Read
  Out1 : Outport  VectorParamsAs1DForOutWhenUnconnected=off
  wires:
  __CoreLabelRead/1(Out1) -> Out1/1

== system Timers_Basic/PLC Controller Suite/__Logic/Task/Program/__Logic/XIC1/BlockEnableRead/__CoreLabelRead ==
  DataRead : DataStoreRead  DataStoreName=x_PLCLabel__s4_3653__Block_Enable  IndexOptions=Index vector (dialog)  Indices=1  OutputSizes=1
  Out1 : Outport  VectorParamsAs1DForOutWhenUnconnected=off
  wires:
  DataRead/1 -> Out1/1

== system Timers_Basic/PLC Controller Suite/__Logic/Task/Program/__Logic/XIC1/Instruction_Enable/__CoreVarRead ==
  DataRead : DataStoreRead  DataStoreName=xxx_PLC_VAR_T  DataStoreElements=xxx_PLC_VAR_T.DN  IndexOptions=Index vector (dialog)  Indices=1  OutputSizes=1
  y : Outport  VectorParamsAs1DForOutWhenUnconnected=off
  wires:
  DataRead/1 -> y/1

== system Timers_Basic/PLC Controller Suite/__Logic/Task/Program/__Logic/XIC1/RungInOverride/ForceRungInFalseRead ==
  __CoreLabelRead : Subsystem  Tag=CoreVarReadBlock  DisableCoverage=on  TreatAsAtomicUnit=on  mask{PLCBlockType=CoreLabelRead}
      mask init:
      | slplc.callbacks.initRoutineLabelRead(gcb);
      mask Help: web([docroot '/plccoder/ref/__corelabelread' '.html']);
      mask DialogControl PLCBlockTitle Prompt: Core Label Read
  Out1 : Outport  VectorParamsAs1DForOutWhenUnconnected=off
  wires:
  __CoreLabelRead/1(Out1) -> Out1/1

== system Timers_Basic/PLC Controller Suite/__Logic/Task/Program/__Logic/OTE/Instruction_Enable/Initialize Function/__CoreVarWrite ==
  u : Inport
  DataWrite : DataStoreWrite  DataStoreName=xxx_PLC_VAR_Out  IndexOptions=Index vector (dialog)  Indices=1  OutputSizes=1
  wires:
  u/1 -> DataWrite/1

== system Timers_Basic/PLC Controller Suite/__Logic/Task/Program/__Logic/OTE/Instruction_Enable/Rung-condition is false/__CoreVarWrite ==
  u : Inport
  DataWrite : DataStoreWrite  DataStoreName=xxx_PLC_VAR_Out  IndexOptions=Index vector (dialog)  Indices=1  OutputSizes=1
  wires:
  u/1 -> DataWrite/1

== system Timers_Basic/PLC Controller Suite/__Logic/Task/Program/__Logic/OTE/Instruction_Enable/Rung-condition-in is true/__CoreVarWrite ==
  u : Inport
  DataWrite : DataStoreWrite  DataStoreName=xxx_PLC_VAR_Out  IndexOptions=Index vector (dialog)  Indices=1  OutputSizes=1
  wires:
  u/1 -> DataWrite/1

== system Timers_Basic/PLC Controller Suite/__Logic/Task/Program/__Logic/OTE/RungInOverride/ForceRungInFalseRead/__CoreLabelRead ==
  DataRead : DataStoreRead  DataStoreName=x_PLCLabel__s4_3653__Force_RungIn_False  IndexOptions=Index vector (dialog)  Indices=1  OutputSizes=1
  Out1 : Outport  VectorParamsAs1DForOutWhenUnconnected=off
  wires:
  DataRead/1 -> Out1/1

== system Timers_Basic/PLC Controller Suite/__Logic/Task/Program/__Logic/TON/Instruction_Enable/Initialize Function/VarWrite ==
  In1 : Inport
  __CoreVarWrite : Subsystem  Tag=CoreVarWriteBlock  DisableCoverage=on  TreatAsAtomicUnit=on  mask{PLCBlockType=CoreVarWrite}
      mask init:
      | slplc.callbacks.initCoreVariable(gcb, 'write');
      mask Help: web([docroot '/plccoder/ref/__corevarwrite' '.html']);
      mask DialogControl PLCBlockTitle Prompt: Core Variable Write
  wires:
  In1/1 -> __CoreVarWrite/1(u)

== system Timers_Basic/PLC Controller Suite/__Logic/Task/Program/__Logic/TON/Instruction_Enable/Initialize Function/VarWrite1 ==
  In1 : Inport
  __CoreVarWrite : Subsystem  Tag=CoreVarWriteBlock  DisableCoverage=on  TreatAsAtomicUnit=on  mask{PLCBlockType=CoreVarWrite}
      mask init:
      | slplc.callbacks.initCoreVariable(gcb, 'write');
      mask Help: web([docroot '/plccoder/ref/__corevarwrite' '.html']);
      mask DialogControl PLCBlockTitle Prompt: Core Variable Write
  wires:
  In1/1 -> __CoreVarWrite/1(u)

== system Timers_Basic/PLC Controller Suite/__Logic/Task/Program/__Logic/TON/Instruction_Enable/Initialize Function/VarWrite2 ==
  In1 : Inport
  __CoreVarWrite : Subsystem  Tag=CoreVarWriteBlock  DisableCoverage=on  TreatAsAtomicUnit=on  mask{PLCBlockType=CoreVarWrite}
      mask init:
      | slplc.callbacks.initCoreVariable(gcb, 'write');
      mask Help: web([docroot '/plccoder/ref/__corevarwrite' '.html']);
      mask DialogControl PLCBlockTitle Prompt: Core Variable Write
  wires:
  In1/1 -> __CoreVarWrite/1(u)

== system Timers_Basic/PLC Controller Suite/__Logic/Task/Program/__Logic/TON/Instruction_Enable/Initialize Function/VarWrite3 ==
  In1 : Inport
  __CoreVarWrite : Subsystem  Tag=CoreVarWriteBlock  DisableCoverage=on  TreatAsAtomicUnit=on  mask{PLCBlockType=CoreVarWrite}
      mask init:
      | slplc.callbacks.initCoreVariable(gcb, 'write');
      mask Help: web([docroot '/plccoder/ref/__corevarwrite' '.html']);
      mask DialogControl PLCBlockTitle Prompt: Core Variable Write
  wires:
  In1/1 -> __CoreVarWrite/1(u)

== system Timers_Basic/PLC Controller Suite/__Logic/Task/Program/__Logic/TON/RungInOverride/ForceRungInFalseRead/__CoreLabelRead ==
  DataRead : DataStoreRead  DataStoreName=x_PLCLabel__s4_3653__Force_RungIn_False  IndexOptions=Index vector (dialog)  Indices=1  OutputSizes=1
  Out1 : Outport  VectorParamsAs1DForOutWhenUnconnected=off
  wires:
  DataRead/1 -> Out1/1
